simulink model "SIMULINK_PID_Tracking"  (R2023b)
settings: Solver=FixedStepAuto  StartTime=0.0  StopTime=sim_end_time  FixedStep=fixed_step_size  RelTol=1e-3
undefined symbols (not defined in the file): a, act_end, b, battery_threshold, bb, draw_gif, droneyeeUAV2_NUM, droneyeeUAV3_NUM, droneyeeUAV4_NUM, droneyeeUAV5_NUM, fixed_step_size, k, KD_x, KD_y, kd_z, KDD_x, KDD_y, KI_x, KI_y, ki_z, KII_x, KII_y, KP_x, KP_y, kp_z, KPP_x, KPP_y, lmt, omega, R, sim_end_time, uav10num, uav1num, uav2num, uav3num, uav4num, uav5num, uav6num, uav7num, uav8num, uav9num, UAV_NUM, Vel_Switch_1, Vel_Switch_10, Vel_Switch_11, Vel_Switch_12, Vel_Switch_13, Vel_Switch_14, Vel_Switch_15, Vel_Switch_16, Vel_Switch_17, Vel_Switch_18, Vel_Switch_19, Vel_Switch_2, Vel_Switch_20, Vel_Switch_3, Vel_Switch_4, Vel_Switch_5, Vel_Switch_6, Vel_Switch_7 ... (+12)
libraries: simulink x120, aerolibanimutils x1
(part 7 of 10)

== system SIMULINK_PID_Tracking/CMD_UAV/CMD3/Subsystem ==
  clock : Inport
  uavstates : Inport  Port=2
  Constant : Constant  Value=uav3num
  MATLAB Function : MATLAB Function  TreatAsAtomicUnit=on
  "xd " : Outport  VectorParamsAs1DForOutWhenUnconnected=off
  yd : Outport  Port=2  VectorParamsAs1DForOutWhenUnconnected=off
  zd : Outport  Port=3  VectorParamsAs1DForOutWhenUnconnected=off
  wires:
  uavstates/1 -> MATLAB Function/4(stas)
  [switch_flag] -> MATLAB Function/3(switch_flag)
  [avo_flag] -> MATLAB Function/7(avo_flag)
  [trj_flag] -> MATLAB Function/5(trj_flag)
  Constant/1 -> MATLAB Function/2(uavnum)
  [form_flag] -> MATLAB Function/6(form_flag)
  clock/1 -> MATLAB Function/1(timestamp)
  MATLAB Function/1(x_) -> "xd "/1
  MATLAB Function/2(y_) -> yd/1
  MATLAB Function/3(z_) -> zd/1

== system SIMULINK_PID_Tracking/CMD_UAV/CMD4/Subsystem ==
  clock : Inport
  uavstates : Inport  Port=2
  Constant : Constant  Value=uav4num
  MATLAB Function : MATLAB Function  TreatAsAtomicUnit=on
  "xd " : Outport  VectorParamsAs1DForOutWhenUnconnected=off
  yd : Outport  Port=2  VectorParamsAs1DForOutWhenUnconnected=off
  zd : Outport  Port=3  VectorParamsAs1DForOutWhenUnconnected=off
  wires:
  uavstates/1 -> MATLAB Function/4(stas)
  [switch_flag] -> MATLAB Function/3(switch_flag)
  [avo_flag] -> MATLAB Function/7(avo_flag)
  [trj_flag] -> MATLAB Function/5(trj_flag)
  Constant/1 -> MATLAB Function/2(uavnum)
  [form_flag] -> MATLAB Function/6(form_flag)
  clock/1 -> MATLAB Function/1(timestamp)
  MATLAB Function/1(x_) -> "xd "/1
  MATLAB Function/2(y_) -> yd/1
  MATLAB Function/3(z_) -> zd/1

== system SIMULINK_PID_Tracking/CMD_UAV/CMD5/Subsystem ==
  clock : Inport
  uavstates : Inport  Port=2
  Constant : Constant  Value=uav5num
  MATLAB Function : MATLAB Function  TreatAsAtomicUnit=on
  "xd " : Outport  VectorParamsAs1DForOutWhenUnconnected=off
  yd : Outport  Port=2  VectorParamsAs1DForOutWhenUnconnected=off
  zd : Outport  Port=3  VectorParamsAs1DForOutWhenUnconnected=off
  wires:
  uavstates/1 -> MATLAB Function/4(stas)
  [switch_flag] -> MATLAB Function/3(switch_flag)
  [avo_flag] -> MATLAB Function/7(avo_flag)
  [trj_flag] -> MATLAB Function/5(trj_flag)
  Constant/1 -> MATLAB Function/2(uavnum)
  [form_flag] -> MATLAB Function/6(form_flag)
  clock/1 -> MATLAB Function/1(timestamp)
  MATLAB Function/1(x_) -> "xd "/1
  MATLAB Function/2(y_) -> yd/1
  MATLAB Function/3(z_) -> zd/1

== system SIMULINK_PID_Tracking/CMD_UAV/CMD6/Subsystem ==
  clock : Inport
  uavstates : Inport  Port=2
  Constant : Constant  Value=uav6num
  MATLAB Function : MATLAB Function  TreatAsAtomicUnit=on
  "xd " : Outport  VectorParamsAs1DForOutWhenUnconnected=off
  yd : Outport  Port=2  VectorParamsAs1DForOutWhenUnconnected=off
  zd : Outport  Port=3  VectorParamsAs1DForOutWhenUnconnected=off
  wires:
  MATLAB Function/1(x_) -> "xd "/1
  MATLAB Function/2(y_) -> yd/1
  MATLAB Function/3(z_) -> zd/1
  clock/1 -> MATLAB Function/1(timestamp)
  Constant/1 -> MATLAB Function/2(uavnum)
  [switch_flag] -> MATLAB Function/3(switch_flag)
  uavstates/1 -> MATLAB Function/4(stas)
  [trj_flag] -> MATLAB Function/5(trj_flag)
  [form_flag] -> MATLAB Function/6(form_flag)
  [avo_flag] -> MATLAB Function/7(avo_flag)

== system SIMULINK_PID_Tracking/CMD_UAV/CMD7/Subsystem ==
  clock : Inport
  uavstates : Inport  Port=2
  Constant : Constant  Value=uav7num
  MATLAB Function : MATLAB Function  TreatAsAtomicUnit=on
  "xd " : Outport  VectorParamsAs1DForOutWhenUnconnected=off
  yd : Outport  Port=2  VectorParamsAs1DForOutWhenUnconnected=off
  zd : Outport  Port=3  VectorParamsAs1DForOutWhenUnconnected=off
  wires:
  uavstates/1 -> MATLAB Function/4(stas)
  [switch_flag] -> MATLAB Function/3(switch_flag)
  [avo_flag] -> MATLAB Function/7(avo_flag)
  [trj_flag] -> MATLAB Function/5(trj_flag)
  Constant/1 -> MATLAB Function/2(uavnum)
  [form_flag] -> MATLAB Function/6(form_flag)
  clock/1 -> MATLAB Function/1(timestamp)
  MATLAB Function/1(x_) -> "xd "/1
  MATLAB Function/2(y_) -> yd/1
  MATLAB Function/3(z_) -> zd/1

== system SIMULINK_PID_Tracking/CMD_UAV/CMD8/Subsystem ==
  clock : Inport
  uavstates : Inport  Port=2
  Constant : Constant  Value=uav8num
  MATLAB Function : MATLAB Function  TreatAsAtomicUnit=on
  "xd " : Outport  VectorParamsAs1DForOutWhenUnconnected=off
  yd : Outport  Port=2  VectorParamsAs1DForOutWhenUnconnected=off
  zd : Outport  Port=3  VectorParamsAs1DForOutWhenUnconnected=off
  wires:
  MATLAB Function/1(x_) -> "xd "/1
  MATLAB Function/2(y_) -> yd/1
  MATLAB Function/3(z_) -> zd/1
  clock/1 -> MATLAB Function/1(timestamp)
  Constant/1 -> MATLAB Function/2(uavnum)
  [switch_flag] -> MATLAB Function/3(switch_flag)
  uavstates/1 -> MATLAB Function/4(stas)
  [trj_flag] -> MATLAB Function/5(trj_flag)
  [form_flag] -> MATLAB Function/6(form_flag)
  [avo_flag] -> MATLAB Function/7(avo_flag)

== system SIMULINK_PID_Tracking/CMD_UAV/CMD9/Subsystem ==
  clock : Inport
  uavstates : Inport  Port=2
  Constant : Constant  Value=uav9num
  MATLAB Function : MATLAB Function  TreatAsAtomicUnit=on
  "xd " : Outport  VectorParamsAs1DForOutWhenUnconnected=off
  yd : Outport  Port=2  VectorParamsAs1DForOutWhenUnconnected=off
  zd : Outport  Port=3  VectorParamsAs1DForOutWhenUnconnected=off
  wires:
  uavstates/1 -> MATLAB Function/4(stas)
  [switch_flag] -> MATLAB Function/3(switch_flag)
  [avo_flag] -> MATLAB Function/7(avo_flag)
  [trj_flag] -> MATLAB Function/5(trj_flag)
  Constant/1 -> MATLAB Function/2(uavnum)
  [form_flag] -> MATLAB Function/6(form_flag)
  clock/1 -> MATLAB Function/1(timestamp)
  MATLAB Function/1(x_) -> "xd "/1
  MATLAB Function/2(y_) -> yd/1
  MATLAB Function/3(z_) -> zd/1

== system SIMULINK_PID_Tracking/CMD_car1/CMD1/Subsystem ==
  clock : Inport
  uavstates : Inport  Port=2
  Constant : Constant  Value=uav1num
  MATLAB Function : MATLAB Function  TreatAsAtomicUnit=on
  "xd " : Outport  VectorParamsAs1DForOutWhenUnconnected=off
  yd : Outport  Port=2  VectorParamsAs1DForOutWhenUnconnected=off
  zd : Outport  Port=3  VectorParamsAs1DForOutWhenUnconnected=off
  wires:
  MATLAB Function/1(x_) -> "xd "/1
  MATLAB Function/2(y_) -> yd/1
  MATLAB Function/3(z_) -> zd/1
  clock/1 -> MATLAB Function/1(timestamp)
  Constant/1 -> MATLAB Function/2(uavnum)
  [switch_flag] -> MATLAB Function/3(switch_flag)
  uavstates/1 -> MATLAB Function/4(stas)
  [trj_flag] -> MATLAB Function/5(trj_flag)
  [form_flag] -> MATLAB Function/6(form_flag)
  [avo_flag] -> MATLAB Function/7(avo_flag)

== system SIMULINK_PID_Tracking/CMD_car1/CMD10/Subsystem ==
  clock : Inport
  uavstates : Inport  Port=2
  Constant : Constant  Value=uav10num
  Goto : Goto  Commented=on  GotoTag=trj_flag  TagVisibility=global
  Goto1 : Goto  Commented=on  GotoTag=form_flag  TagVisibility=global
  Goto2 : Goto  Commented=on  GotoTag=avo_flag  TagVisibility=global
  MATLAB Function : MATLAB Function  TreatAsAtomicUnit=on
  轨迹 : Constant  Commented=on
  避障 : Constant  Commented=on  Value=0
  队形 : Constant  Commented=on
  "xd " : Outport  VectorParamsAs1DForOutWhenUnconnected=off
  yd : Outport  Port=2  VectorParamsAs1DForOutWhenUnconnected=off
  zd : Outport  Port=3  VectorParamsAs1DForOutWhenUnconnected=off
  wires:
  MATLAB Function/1(x_) -> "xd "/1
  MATLAB Function/2(y_) -> yd/1
  MATLAB Function/3(z_) -> zd/1
  clock/1 -> MATLAB Function/1(timestamp)
  Constant/1 -> MATLAB Function/2(uavnum)
  [switch_flag] -> MATLAB Function/3(switch_flag)
  uavstates/1 -> MATLAB Function/4(stas)
  轨迹/1 -> Goto/1
  队形/1 -> Goto1/1
  避障/1 -> Goto2/1
  [trj_flag] -> MATLAB Function/5(trj_flag)
  [form_flag] -> MATLAB Function/6(form_flag)
  [avo_flag] -> MATLAB Function/7(avo_flag)

== system SIMULINK_PID_Tracking/CMD_car1/CMD2/Subsystem ==
  clock : Inport
  uavstates : Inport  Port=2
  Constant : Constant  Value=uav2num
  MATLAB Function : MATLAB Function  TreatAsAtomicUnit=on
  "xd " : Outport  VectorParamsAs1DForOutWhenUnconnected=off
  yd : Outport  Port=2  VectorParamsAs1DForOutWhenUnconnected=off
  zd : Outport  Port=3  VectorParamsAs1DForOutWhenUnconnected=off
  wires:
  uavstates/1 -> MATLAB Function/4(stas)
  [switch_flag] -> MATLAB Function/3(switch_flag)
  [avo_flag] -> MATLAB Function/7(avo_flag)
  [trj_flag] -> MATLAB Function/5(trj_flag)
  Constant/1 -> MATLAB Function/2(uavnum)
  [form_flag] -> MATLAB Function/6(form_flag)
  clock/1 -> MATLAB Function/1(timestamp)
  MATLAB Function/1(x_) -> "xd "/1
  MATLAB Function/3(z_) -> zd/1
  MATLAB Function/2(y_) -> yd/1

== system SIMULINK_PID_Tracking/CMD_car1/CMD3/Subsystem ==
  clock : Inport
  uavstates : Inport  Port=2
  Constant : Constant  Value=uav3num
  MATLAB Function : MATLAB Function  TreatAsAtomicUnit=on
  "xd " : Outport  VectorParamsAs1DForOutWhenUnconnected=off
  yd : Outport  Port=2  VectorParamsAs1DForOutWhenUnconnected=off
  zd : Outport  Port=3  VectorParamsAs1DForOutWhenUnconnected=off
  wires:
  uavstates/1 -> MATLAB Function/4(stas)
  [switch_flag] -> MATLAB Function/3(switch_flag)
  [avo_flag] -> MATLAB Function/7(avo_flag)
  [trj_flag] -> MATLAB Function/5(trj_flag)
  Constant/1 -> MATLAB Function/2(uavnum)
  [form_flag] -> MATLAB Function/6(form_flag)
  clock/1 -> MATLAB Function/1(timestamp)
  MATLAB Function/1(x_) -> "xd "/1
  MATLAB Function/2(y_) -> yd/1
  MATLAB Function/3(z_) -> zd/1

== system SIMULINK_PID_Tracking/CMD_car1/CMD4/Subsystem ==
  clock : Inport
  uavstates : Inport  Port=2
  Constant : Constant  Value=uav4num
  MATLAB Function : MATLAB Function  TreatAsAtomicUnit=on
  "xd " : Outport  VectorParamsAs1DForOutWhenUnconnected=off
  yd : Outport  Port=2  VectorParamsAs1DForOutWhenUnconnected=off
  zd : Outport  Port=3  VectorParamsAs1DForOutWhenUnconnected=off
  wires:
  uavstates/1 -> MATLAB Function/4(stas)
  [switch_flag] -> MATLAB Function/3(switch_flag)
  [avo_flag] -> MATLAB Function/7(avo_flag)
  [trj_flag] -> MATLAB Function/5(trj_flag)
  Constant/1 -> MATLAB Function/2(uavnum)
  [form_flag] -> MATLAB Function/6(form_flag)
  clock/1 -> MATLAB Function/1(timestamp)
  MATLAB Function/1(x_) -> "xd "/1
  MATLAB Function/2(y_) -> yd/1
  MATLAB Function/3(z_) -> zd/1

== system SIMULINK_PID_Tracking/CMD_car1/CMD5/Subsystem ==
  clock : Inport
  uavstates : Inport  Port=2
  Constant : Constant  Value=uav5num
  MATLAB Function : MATLAB Function  TreatAsAtomicUnit=on
  "xd " : Outport  VectorParamsAs1DForOutWhenUnconnected=off
  yd : Outport  Port=2  VectorParamsAs1DForOutWhenUnconnected=off
  zd : Outport  Port=3  VectorParamsAs1DForOutWhenUnconnected=off
  wires:
  uavstates/1 -> MATLAB Function/4(stas)
  [switch_flag] -> MATLAB Function/3(switch_flag)
  [avo_flag] -> MATLAB Function/7(avo_flag)
  [trj_flag] -> MATLAB Function/5(trj_flag)
  Constant/1 -> MATLAB Function/2(uavnum)
  [form_flag] -> MATLAB Function/6(form_flag)
  clock/1 -> MATLAB Function/1(timestamp)
  MATLAB Function/1(x_) -> "xd "/1
  MATLAB Function/2(y_) -> yd/1
  MATLAB Function/3(z_) -> zd/1

== system SIMULINK_PID_Tracking/CMD_car1/CMD6/Subsystem ==
  clock : Inport
  uavstates : Inport  Port=2
  Constant : Constant  Value=uav6num
  MATLAB Function : MATLAB Function  TreatAsAtomicUnit=on
  "xd " : Outport  VectorParamsAs1DForOutWhenUnconnected=off
  yd : Outport  Port=2  VectorParamsAs1DForOutWhenUnconnected=off
  zd : Outport  Port=3  VectorParamsAs1DForOutWhenUnconnected=off
  wires:
  MATLAB Function/1(x_) -> "xd "/1
  MATLAB Function/2(y_) -> yd/1
  MATLAB Function/3(z_) -> zd/1
  clock/1 -> MATLAB Function/1(timestamp)
  Constant/1 -> MATLAB Function/2(uavnum)
  [switch_flag] -> MATLAB Function/3(switch_flag)
  uavstates/1 -> MATLAB Function/4(stas)
  [trj_flag] -> MATLAB Function/5(trj_flag)
  [form_flag] -> MATLAB Function/6(form_flag)
  [avo_flag] -> MATLAB Function/7(avo_flag)

== system SIMULINK_PID_Tracking/CMD_car1/CMD7/Subsystem ==
  clock : Inport
  uavstates : Inport  Port=2
  Constant : Constant  Value=uav7num
  MATLAB Function : MATLAB Function  TreatAsAtomicUnit=on
  "xd " : Outport  VectorParamsAs1DForOutWhenUnconnected=off
  yd : Outport  Port=2  VectorParamsAs1DForOutWhenUnconnected=off
  zd : Outport  Port=3  VectorParamsAs1DForOutWhenUnconnected=off
  wires:
  uavstates/1 -> MATLAB Function/4(stas)
  [switch_flag] -> MATLAB Function/3(switch_flag)
  [avo_flag] -> MATLAB Function/7(avo_flag)
  [trj_flag] -> MATLAB Function/5(trj_flag)
  Constant/1 -> MATLAB Function/2(uavnum)
  [form_flag] -> MATLAB Function/6(form_flag)
  clock/1 -> MATLAB Function/1(timestamp)
  MATLAB Function/1(x_) -> "xd "/1
  MATLAB Function/2(y_) -> yd/1
  MATLAB Function/3(z_) -> zd/1

== system SIMULINK_PID_Tracking/CMD_car1/CMD8/Subsystem ==
  clock : Inport
  uavstates : Inport  Port=2
  Constant : Constant  Value=uav8num
  MATLAB Function : MATLAB Function  TreatAsAtomicUnit=on
  "xd " : Outport  VectorParamsAs1DForOutWhenUnconnected=off
  yd : Outport  Port=2  VectorParamsAs1DForOutWhenUnconnected=off
  zd : Outport  Port=3  VectorParamsAs1DForOutWhenUnconnected=off
  wires:
  MATLAB Function/1(x_) -> "xd "/1
  MATLAB Function/2(y_) -> yd/1
  MATLAB Function/3(z_) -> zd/1
  clock/1 -> MATLAB Function/1(timestamp)
  Constant/1 -> MATLAB Function/2(uavnum)
  [switch_flag] -> MATLAB Function/3(switch_flag)
  uavstates/1 -> MATLAB Function/4(stas)
  [trj_flag] -> MATLAB Function/5(trj_flag)
  [form_flag] -> MATLAB Function/6(form_flag)
  [avo_flag] -> MATLAB Function/7(avo_flag)

== system SIMULINK_PID_Tracking/CMD_car1/CMD9/Subsystem ==
  clock : Inport
  uavstates : Inport  Port=2
  Constant : Constant  Value=uav9num
  MATLAB Function : MATLAB Function  TreatAsAtomicUnit=on
  "xd " : Outport  VectorParamsAs1DForOutWhenUnconnected=off
  yd : Outport  Port=2  VectorParamsAs1DForOutWhenUnconnected=off
  zd : Outport  Port=3  VectorParamsAs1DForOutWhenUnconnected=off
  wires:
  uavstates/1 -> MATLAB Function/4(stas)
  [switch_flag] -> MATLAB Function/3(switch_flag)
  [avo_flag] -> MATLAB Function/7(avo_flag)
  [trj_flag] -> MATLAB Function/5(trj_flag)
  Constant/1 -> MATLAB Function/2(uavnum)
  [form_flag] -> MATLAB Function/6(form_flag)
  clock/1 -> MATLAB Function/1(timestamp)
  MATLAB Function/1(x_) -> "xd "/1
  MATLAB Function/2(y_) -> yd/1
  MATLAB Function/3(z_) -> zd/1

== system SIMULINK_PID_Tracking/control system_UAV/Baseline Controller1/Heading controller ==
  yaw_e (rad) : Inport
  yaw_d. (rad) : Inport  Port=2
  Integrator Limited : Integrator  Commented=on  LimitOutput=on  UpperSaturationLimit=0.3  LowerSaturationLimit=-0.3
  Ki : Gain  Commented=on  Gain=0.01
  Sum1 : Sum  Inputs=|-+
  Sum2 : Sum  Inputs=|++
  proportional control gain - yaw : Gain  Gain=0.2
  yaw_rate_d. (rad/s) : Outport  VectorParamsAs1DForOutWhenUnconnected=off
  wires:
  Sum1/1 -> Ki/1, proportional control gain - yaw/1
  yaw_e (rad)/1 -> Sum1/1
  yaw_d. (rad)/1 -> Sum1/2
  proportional control gain - yaw/1 -> Sum2/1
  Integrator Limited/1 -> Sum2/2
  Ki/1 -> Integrator Limited/1
  Sum2/1 -> yaw_rate_d. (rad/s)/1

== system SIMULINK_PID_Tracking/control system_UAV/Baseline Controller1/Height controller  ==
  Z_d. (m) : Inport
  Z_e (m) : Inport  Port=2
  V_z : Inport  Port=3
  Discrete Derivative1 : simulink/Discrete/Discrete Derivative  gainval=1.0  ICPrevScaledInput=0.0  OutMin=[]  OutMax=[]  OutDataType=fixdt(1, 16)  OutScaling=2^-10  DoSatur=off
  Integrator Limited : Integrator  LimitOutput=on  UpperSaturationLimit=0.1  LowerSaturationLimit=-0.1
  Kd : Gain  Gain=kd_z
  Ki : Gain  Gain=ki_z
  Kp : Gain  Gain=kp_z
  Sum2 : Sum  Inputs=+++
  Sum3 : Sum  Inputs=|-+
  Z_velocity_d (m/s) : Outport  VectorParamsAs1DForOutWhenUnconnected=off
  wires:
  Sum3/1 -> Discrete Derivative1/1, Ki/1, Kp/1
  Z_e (m)/1 -> Sum3/1
  Discrete Derivative1/1 -> Kd/1
  Sum2/1 -> Z_velocity_d (m/s)/1
  Kp/1 -> Sum2/2
  Kd/1 -> Sum2/3
  Ki/1 -> Integrator Limited/1
  Integrator Limited/1 -> Sum2/1
  Z_d. (m)/1 -> Sum3/2

== system SIMULINK_PID_Tracking/control system_UAV/Baseline Controller1/Position controller ==
  X_e (m) : Inport
  Y_e (m) : Inport  Port=2
  X_d (m) : Inport  Port=3
  Y_d (m) : Inport  Port=4
  Discrete Derivative1 : simulink/Discrete/Discrete Derivative  gainval=1.0  ICPrevScaledInput=0.0  OutMin=[]  OutMax=[]  OutDataType=fixdt(1, 16)  OutScaling=2^-10  DoSatur=off
  Discrete Derivative2 : simulink/Discrete/Discrete Derivative  gainval=1.0  ICPrevScaledInput=0.0  OutMin=[]  OutMax=[]  OutDataType=fixdt(1, 16)  OutScaling=2^-10  DoSatur=off
  Integrator Limited : Integrator  LimitOutput=on  UpperSaturationLimit=0.4  LowerSaturationLimit=-0.4
  Integrator Limited1 : Integrator  LimitOutput=on  UpperSaturationLimit=0.4  LowerSaturationLimit=-0.4
  Kd : Gain  Gain=KD_x
  Kd1 : Gain  Gain=KD_y
  Kp : Gain  Gain=KP_x
  Kp1 : Gain  Gain=KI_x
  Kp2 : Gain  Gain=KP_y
  Kp3 : Gain  Gain=KI_y
  Mux : Mux  Inputs=2
  Sum2 : Sum  Inputs=+++
  Sum3 : Sum  Inputs=|-+
  Sum5 : Sum  Inputs=+++
  Sum6 : Sum  Inputs=|-+
  uxy : Outport  VectorParamsAs1DForOutWhenUnconnected=off
  wires:
  Sum5/1 -> Mux/2
  Discrete Derivative1/1 -> Kd/1
  Kp2/1 -> Sum5/2
  Sum3/1 -> Discrete Derivative1/1, Kp/1, Kp1/1
  Discrete Derivative2/1 -> Kd1/1
  X_d (m)/1 -> Sum3/2
  Integrator Limited/1 -> Sum2/1
  Y_d (m)/1 -> Sum6/2
  Kp3/1 -> Integrator Limited1/1
  Kp1/1 -> Integrator Limited/1
  Kd1/1 -> Sum5/3
  Mux/1 -> uxy/1
  Kp/1 -> Sum2/2
  X_e (m)/1 -> Sum3/1
  Integrator Limited1/1 -> Sum5/1
  Sum2/1 -> Mux/1
  Kd/1 -> Sum2/3
  Y_e (m)/1 -> Sum6/1
  Sum6/1 -> Discrete Derivative2/1, Kp2/1, Kp3/1

== system SIMULINK_PID_Tracking/control system_UAV/Baseline Controller10/Heading controller ==
  yaw_e (rad) : Inport
  yaw_d. (rad) : Inport  Port=2
  Integrator Limited : Integrator  Commented=on  LimitOutput=on  UpperSaturationLimit=0.3  LowerSaturationLimit=-0.3
  Ki : Gain  Commented=on  Gain=0.01
  Sum1 : Sum  Inputs=|-+
  Sum2 : Sum  Inputs=|++
  proportional control gain - yaw : Gain  Gain=0.2
  yaw_rate_d. (rad/s) : Outport  VectorParamsAs1DForOutWhenUnconnected=off
  wires:
  Sum1/1 -> Ki/1, proportional control gain - yaw/1
  yaw_e (rad)/1 -> Sum1/1
  yaw_d. (rad)/1 -> Sum1/2
  proportional control gain - yaw/1 -> Sum2/1
  Integrator Limited/1 -> Sum2/2
  Ki/1 -> Integrator Limited/1
  Sum2/1 -> yaw_rate_d. (rad/s)/1

== system SIMULINK_PID_Tracking/control system_UAV/Baseline Controller10/Height controller  ==
  Z_d. (m) : Inport
  Z_e (m) : Inport  Port=2
  V_z : Inport  Port=3
  Discrete Derivative1 : simulink/Discrete/Discrete Derivative  gainval=1.0  ICPrevScaledInput=0.0  OutMin=[]  OutMax=[]  OutDataType=fixdt(1, 16)  OutScaling=2^-10  DoSatur=off
  Integrator Limited : Integrator  LimitOutput=on  UpperSaturationLimit=0.1  LowerSaturationLimit=-0.1
  Kd : Gain  Gain=kd_z
  Ki : Gain  Gain=ki_z
  Kp : Gain  Gain=kp_z
  Sum2 : Sum  Inputs=+++
  Sum3 : Sum  Inputs=|-+
  Z_velocity_d (m/s) : Outport  VectorParamsAs1DForOutWhenUnconnected=off
  wires:
  Sum3/1 -> Discrete Derivative1/1, Ki/1, Kp/1
  Z_e (m)/1 -> Sum3/1
  Discrete Derivative1/1 -> Kd/1
  Sum2/1 -> Z_velocity_d (m/s)/1
  Kp/1 -> Sum2/2
  Kd/1 -> Sum2/3
  Ki/1 -> Integrator Limited/1
  Integrator Limited/1 -> Sum2/1
  Z_d. (m)/1 -> Sum3/2

== system SIMULINK_PID_Tracking/control system_UAV/Baseline Controller10/Position controller ==
  X_e (m) : Inport
  Y_e (m) : Inport  Port=2
  X_d (m) : Inport  Port=3
  Y_d (m) : Inport  Port=4
  Discrete Derivative1 : simulink/Discrete/Discrete Derivative  gainval=1.0  ICPrevScaledInput=0.0  OutMin=[]  OutMax=[]  OutDataType=fixdt(1, 16)  OutScaling=2^-10  DoSatur=off
  Discrete Derivative2 : simulink/Discrete/Discrete Derivative  gainval=1.0  ICPrevScaledInput=0.0  OutMin=[]  OutMax=[]  OutDataType=fixdt(1, 16)  OutScaling=2^-10  DoSatur=off
  Integrator Limited : Integrator  LimitOutput=on  UpperSaturationLimit=0.5  LowerSaturationLimit=-0.5
  Integrator Limited1 : Integrator  LimitOutput=on  UpperSaturationLimit=0.5  LowerSaturationLimit=-0.5
  Kd : Gain  Gain=KD_x
  Kd1 : Gain  Gain=KD_y
  Kp : Gain  Gain=KP_x
  Kp1 : Gain  Gain=KI_x
  Kp2 : Gain  Gain=KP_y
  Kp3 : Gain  Gain=KI_y
  Mux : Mux  Inputs=2
  Scope : Scope
  Scope1 : Scope
  Sum2 : Sum  Inputs=+++
  Sum3 : Sum  Inputs=|-+
  Sum5 : Sum  Inputs=+++
  Sum6 : Sum  Inputs=|-+
  uxy : Outport  VectorParamsAs1DForOutWhenUnconnected=off
  wires:
  X_e (m)/1 -> Sum3/1
  Integrator Limited/1 -> Sum2/1
  Sum2/1 -> Mux/1, Scope/1
  Kp1/1 -> Integrator Limited/1
  Kp/1 -> Sum2/2
  Kp2/1 -> Sum5/2
  Y_e (m)/1 -> Sum6/1
  Integrator Limited1/1 -> Sum5/1
  Sum5/1 -> Mux/2, Scope1/1
  Kp3/1 -> Integrator Limited1/1
  Mux/1 -> uxy/1
  X_d (m)/1 -> Sum3/2
  Discrete Derivative1/1 -> Kd/1
  Sum3/1 -> Discrete Derivative1/1, Kp/1, Kp1/1
  Y_d (m)/1 -> Sum6/2
  Sum6/1 -> Discrete Derivative2/1, Kp2/1, Kp3/1
  Kd1/1 -> Sum5/3
  Discrete Derivative2/1 -> Kd1/1
  Kd/1 -> Sum2/3

== system SIMULINK_PID_Tracking/control system_UAV/Baseline Controller2/Heading controller ==
  yaw_e (rad) : Inport
  yaw_d. (rad) : Inport  Port=2
  Integrator Limited : Integrator  Commented=on  LimitOutput=on  UpperSaturationLimit=0.3  LowerSaturationLimit=-0.3
  Ki : Gain  Commented=on  Gain=0.01
  Sum1 : Sum  Inputs=|-+
  Sum2 : Sum  Inputs=|++
  proportional control gain - yaw : Gain  Gain=0.2
  yaw_rate_d. (rad/s) : Outport  VectorParamsAs1DForOutWhenUnconnected=off
  wires:
  Sum2/1 -> yaw_rate_d. (rad/s)/1
  Ki/1 -> Integrator Limited/1
  Integrator Limited/1 -> Sum2/2
  proportional control gain - yaw/1 -> Sum2/1
  yaw_d. (rad)/1 -> Sum1/2
  yaw_e (rad)/1 -> Sum1/1
  Sum1/1 -> proportional control gain - yaw/1, Ki/1

== system SIMULINK_PID_Tracking/control system_UAV/Baseline Controller2/Height controller  ==
  Z_d. (m) : Inport
  Z_e (m) : Inport  Port=2
  V_z : Inport  Port=3
  Discrete Derivative1 : simulink/Discrete/Discrete Derivative  gainval=1.0  ICPrevScaledInput=0.0  OutMin=[]  OutMax=[]  OutDataType=fixdt(1, 16)  OutScaling=2^-10  DoSatur=off
  Integrator Limited : Integrator  LimitOutput=on  UpperSaturationLimit=0.1  LowerSaturationLimit=-0.1
  Kd : Gain  Gain=kd_z
  Ki : Gain  Gain=ki_z
  Kp : Gain  Gain=kp_z
  Sum2 : Sum  Inputs=+++
  Sum3 : Sum  Inputs=|-+
  Z_velocity_d (m/s) : Outport  VectorParamsAs1DForOutWhenUnconnected=off
  wires:
  Sum3/1 -> Discrete Derivative1/1, Ki/1, Kp/1
  Z_e (m)/1 -> Sum3/1
  Discrete Derivative1/1 -> Kd/1
  Sum2/1 -> Z_velocity_d (m/s)/1
  Kp/1 -> Sum2/2
  Kd/1 -> Sum2/3
  Ki/1 -> Integrator Limited/1
  Integrator Limited/1 -> Sum2/1
  Z_d. (m)/1 -> Sum3/2

== system SIMULINK_PID_Tracking/control system_UAV/Baseline Controller2/Position controller ==
  X_e (m) : Inport
  Y_e (m) : Inport  Port=2
  X_d (m) : Inport  Port=3
  Y_d (m) : Inport  Port=4
  Discrete Derivative1 : simulink/Discrete/Discrete Derivative  gainval=1.0  ICPrevScaledInput=0.0  OutMin=[]  OutMax=[]  OutDataType=fixdt(1, 16)  OutScaling=2^-10  DoSatur=off
  Discrete Derivative2 : simulink/Discrete/Discrete Derivative  gainval=1.0  ICPrevScaledInput=0.0  OutMin=[]  OutMax=[]  OutDataType=fixdt(1, 16)  OutScaling=2^-10  DoSatur=off
  Integrator Limited : Integrator  LimitOutput=on  UpperSaturationLimit=0.4  LowerSaturationLimit=-0.4
  Integrator Limited1 : Integrator  LimitOutput=on  UpperSaturationLimit=0.4  LowerSaturationLimit=-0.4
  Kd : Gain  Gain=KD_x
  Kd1 : Gain  Gain=KD_y
  Kp : Gain  Gain=KP_x
  Kp1 : Gain  Gain=KI_x
  Kp2 : Gain  Gain=KP_y
  Kp3 : Gain  Gain=KI_y
  Mux : Mux  Inputs=2
  Sum2 : Sum  Inputs=+++
  Sum3 : Sum  Inputs=|-+
  Sum5 : Sum  Inputs=+++
  Sum6 : Sum  Inputs=|-+
  uxy : Outport  VectorParamsAs1DForOutWhenUnconnected=off
  wires:
  Discrete Derivative2/1 -> Kd1/1
  Kd1/1 -> Sum5/3
  Sum6/1 -> Discrete Derivative2/1, Kp2/1, Kp3/1
  Y_d (m)/1 -> Sum6/2
  Kd/1 -> Sum2/3
  Discrete Derivative1/1 -> Kd/1
  Sum3/1 -> Discrete Derivative1/1, Kp1/1, Kp/1
  X_d (m)/1 -> Sum3/2
  Mux/1 -> uxy/1
  Kp3/1 -> Integrator Limited1/1
  Integrator Limited1/1 -> Sum5/1
  Y_e (m)/1 -> Sum6/1
  Kp2/1 -> Sum5/2
  Kp/1 -> Sum2/2
  Kp1/1 -> Integrator Limited/1
  Integrator Limited/1 -> Sum2/1
  X_e (m)/1 -> Sum3/1
  Sum2/1 -> Mux/1
  Sum5/1 -> Mux/2

== system SIMULINK_PID_Tracking/control system_UAV/Baseline Controller3/Heading controller ==
  yaw_e (rad) : Inport
  yaw_d. (rad) : Inport  Port=2
  Integrator Limited : Integrator  Commented=on  LimitOutput=on  UpperSaturationLimit=0.3  LowerSaturationLimit=-0.3
  Ki : Gain  Commented=on  Gain=0.01
  Sum1 : Sum  Inputs=|-+
  Sum2 : Sum  Inputs=|++
  proportional control gain - yaw : Gain  Gain=0.2
  yaw_rate_d. (rad/s) : Outport  VectorParamsAs1DForOutWhenUnconnected=off
  wires:
  Sum1/1 -> Ki/1, proportional control gain - yaw/1
  yaw_e (rad)/1 -> Sum1/1
  yaw_d. (rad)/1 -> Sum1/2
  proportional control gain - yaw/1 -> Sum2/1
  Integrator Limited/1 -> Sum2/2
  Ki/1 -> Integrator Limited/1
  Sum2/1 -> yaw_rate_d. (rad/s)/1

== system SIMULINK_PID_Tracking/control system_UAV/Baseline Controller3/Height controller  ==
  Z_d. (m) : Inport
  Z_e (m) : Inport  Port=2
  V_z : Inport  Port=3
  Discrete Derivative1 : simulink/Discrete/Discrete Derivative  gainval=1.0  ICPrevScaledInput=0.0  OutMin=[]  OutMax=[]  OutDataType=fixdt(1, 16)  OutScaling=2^-10  DoSatur=off
  Integrator Limited : Integrator  LimitOutput=on  UpperSaturationLimit=0.1  LowerSaturationLimit=-0.1
  Kd : Gain  Gain=kd_z
  Ki : Gain  Gain=ki_z
  Kp : Gain  Gain=kp_z
  Sum2 : Sum  Inputs=+++
  Sum3 : Sum  Inputs=|-+
  Z_velocity_d (m/s) : Outport  VectorParamsAs1DForOutWhenUnconnected=off
  wires:
  Sum3/1 -> Discrete Derivative1/1, Ki/1, Kp/1
  Z_e (m)/1 -> Sum3/1
  Discrete Derivative1/1 -> Kd/1
  Sum2/1 -> Z_velocity_d (m/s)/1
  Kp/1 -> Sum2/2
  Kd/1 -> Sum2/3
  Ki/1 -> Integrator Limited/1
  Integrator Limited/1 -> Sum2/1
  Z_d. (m)/1 -> Sum3/2

== system SIMULINK_PID_Tracking/control system_UAV/Baseline Controller3/Position controller ==
  X_e (m) : Inport
  Y_e (m) : Inport  Port=2
  X_d (m) : Inport  Port=3
  Y_d (m) : Inport  Port=4
  Discrete Derivative1 : simulink/Discrete/Discrete Derivative  gainval=1.0  ICPrevScaledInput=0.0  OutMin=[]  OutMax=[]  OutDataType=fixdt(1, 16)  OutScaling=2^-10  DoSatur=off
  Discrete Derivative2 : simulink/Discrete/Discrete Derivative  gainval=1.0  ICPrevScaledInput=0.0  OutMin=[]  OutMax=[]  OutDataType=fixdt(1, 16)  OutScaling=2^-10  DoSatur=off
  Integrator Limited : Integrator  LimitOutput=on  UpperSaturationLimit=0.5  LowerSaturationLimit=-0.5
  Integrator Limited1 : Integrator  LimitOutput=on  UpperSaturationLimit=0.5  LowerSaturationLimit=-0.5
  Kd : Gain  Gain=KD_x
  Kd1 : Gain  Gain=KD_y
  Kp : Gain  Gain=KP_x
  Kp1 : Gain  Gain=KI_x
  Kp2 : Gain  Gain=KP_y
  Kp3 : Gain  Gain=KI_y
  Mux : Mux  Inputs=2
  Sum2 : Sum  Inputs=+++
  Sum3 : Sum  Inputs=|-+
  Sum5 : Sum  Inputs=+++
  Sum6 : Sum  Inputs=|-+
  uxy : Outport  VectorParamsAs1DForOutWhenUnconnected=off
  wires:
  X_e (m)/1 -> Sum3/1
  Integrator Limited/1 -> Sum2/1
  Kp1/1 -> Integrator Limited/1
  Kp/1 -> Sum2/2
  Kp2/1 -> Sum5/2
  Y_e (m)/1 -> Sum6/1
  Integrator Limited1/1 -> Sum5/1
  Kp3/1 -> Integrator Limited1/1
  Mux/1 -> uxy/1
  X_d (m)/1 -> Sum3/2
  Discrete Derivative1/1 -> Kd/1
  Kd/1 -> Sum2/3
  Sum3/1 -> Discrete Derivative1/1, Kp/1, Kp1/1
  Y_d (m)/1 -> Sum6/2
  Sum6/1 -> Discrete Derivative2/1, Kp2/1, Kp3/1
  Kd1/1 -> Sum5/3
  Discrete Derivative2/1 -> Kd1/1
  Sum2/1 -> Mux/1
  Sum5/1 -> Mux/2

== system SIMULINK_PID_Tracking/control system_UAV/Baseline Controller4/Heading controller ==
  yaw_e (rad) : Inport
  yaw_d. (rad) : Inport  Port=2
  Integrator Limited : Integrator  Commented=on  LimitOutput=on  UpperSaturationLimit=0.3  LowerSaturationLimit=-0.3
  Ki : Gain  Commented=on  Gain=0.01
  Sum1 : Sum  Inputs=|-+
  Sum2 : Sum  Inputs=|++
  proportional control gain - yaw : Gain  Gain=0.2
  yaw_rate_d. (rad/s) : Outport  VectorParamsAs1DForOutWhenUnconnected=off
  wires:
  Sum2/1 -> yaw_rate_d. (rad/s)/1
  Ki/1 -> Integrator Limited/1
  Integrator Limited/1 -> Sum2/2
  proportional control gain - yaw/1 -> Sum2/1
  yaw_d. (rad)/1 -> Sum1/2
  yaw_e (rad)/1 -> Sum1/1
  Sum1/1 -> proportional control gain - yaw/1, Ki/1

== system SIMULINK_PID_Tracking/control system_UAV/Baseline Controller4/Height controller  ==
  Z_d. (m) : Inport
  Z_e (m) : Inport  Port=2
  V_z : Inport  Port=3
  Discrete Derivative1 : simulink/Discrete/Discrete Derivative  gainval=1.0  ICPrevScaledInput=0.0  OutMin=[]  OutMax=[]  OutDataType=fixdt(1, 16)  OutScaling=2^-10  DoSatur=off
  Integrator Limited : Integrator  LimitOutput=on  UpperSaturationLimit=0.1  LowerSaturationLimit=-0.1
  Kd : Gain  Gain=kd_z
  Ki : Gain  Gain=ki_z
  Kp : Gain  Gain=kp_z
  Sum2 : Sum  Inputs=+++
  Sum3 : Sum  Inputs=|-+
  Z_velocity_d (m/s) : Outport  VectorParamsAs1DForOutWhenUnconnected=off
  wires:
  Sum3/1 -> Discrete Derivative1/1, Ki/1, Kp/1
  Z_e (m)/1 -> Sum3/1
  Discrete Derivative1/1 -> Kd/1
  Sum2/1 -> Z_velocity_d (m/s)/1
  Kp/1 -> Sum2/2
  Kd/1 -> Sum2/3
  Ki/1 -> Integrator Limited/1
  Integrator Limited/1 -> Sum2/1
  Z_d. (m)/1 -> Sum3/2

== system SIMULINK_PID_Tracking/control system_UAV/Baseline Controller4/Position controller ==
  X_e (m) : Inport
  Y_e (m) : Inport  Port=2
  X_d (m) : Inport  Port=3
  Y_d (m) : Inport  Port=4
  Discrete Derivative1 : simulink/Discrete/Discrete Derivative  gainval=1.0  ICPrevScaledInput=0.0  OutMin=[]  OutMax=[]  OutDataType=fixdt(1, 16)  OutScaling=2^-10  DoSatur=off
  Discrete Derivative2 : simulink/Discrete/Discrete Derivative  gainval=1.0  ICPrevScaledInput=0.0  OutMin=[]  OutMax=[]  OutDataType=fixdt(1, 16)  OutScaling=2^-10  DoSatur=off
  Integrator Limited : Integrator  LimitOutput=on  UpperSaturationLimit=0.5  LowerSaturationLimit=-0.5
  Integrator Limited1 : Integrator  LimitOutput=on  UpperSaturationLimit=0.5  LowerSaturationLimit=-0.5
  Kd : Gain  Gain=KD_x
  Kd1 : Gain  Gain=KD_y
  Kp : Gain  Gain=KP_x
  Kp1 : Gain  Gain=KI_x
  Kp2 : Gain  Gain=KP_y
  Kp3 : Gain  Gain=KI_y
  Mux : Mux  Inputs=2
  Sum2 : Sum  Inputs=+++
  Sum3 : Sum  Inputs=|-+
  Sum5 : Sum  Inputs=+++
  Sum6 : Sum  Inputs=|-+
  uxy : Outport  VectorParamsAs1DForOutWhenUnconnected=off
  wires:
  Discrete Derivative2/1 -> Kd1/1
  Kd1/1 -> Sum5/3
  Sum6/1 -> Discrete Derivative2/1, Kp3/1, Kp2/1
  Y_d (m)/1 -> Sum6/2
  Sum3/1 -> Discrete Derivative1/1, Kp1/1, Kp/1
  Kd/1 -> Sum2/3
  Discrete Derivative1/1 -> Kd/1
  X_d (m)/1 -> Sum3/2
  Mux/1 -> uxy/1
  Kp3/1 -> Integrator Limited1/1
  Integrator Limited1/1 -> Sum5/1
  Y_e (m)/1 -> Sum6/1
  Kp2/1 -> Sum5/2
  Kp/1 -> Sum2/2
  Kp1/1 -> Integrator Limited/1
  Integrator Limited/1 -> Sum2/1
  X_e (m)/1 -> Sum3/1
  Sum5/1 -> Mux/2
  Sum2/1 -> Mux/1

== system SIMULINK_PID_Tracking/control system_UAV/Baseline Controller5/Heading controller ==
  yaw_e (rad) : Inport
  yaw_d. (rad) : Inport  Port=2
  Integrator Limited : Integrator  Commented=on  LimitOutput=on  UpperSaturationLimit=0.3  LowerSaturationLimit=-0.3
  Ki : Gain  Commented=on  Gain=0.01
  Sum1 : Sum  Inputs=|-+
  Sum2 : Sum  Inputs=|++
  proportional control gain - yaw : Gain  Gain=0.2
  yaw_rate_d. (rad/s) : Outport  VectorParamsAs1DForOutWhenUnconnected=off
  wires:
  Sum1/1 -> Ki/1, proportional control gain - yaw/1
  yaw_e (rad)/1 -> Sum1/1
  yaw_d. (rad)/1 -> Sum1/2
  proportional control gain - yaw/1 -> Sum2/1
  Integrator Limited/1 -> Sum2/2
  Ki/1 -> Integrator Limited/1
  Sum2/1 -> yaw_rate_d. (rad/s)/1

== system SIMULINK_PID_Tracking/control system_UAV/Baseline Controller5/Height controller  ==
  Z_d. (m) : Inport
  Z_e (m) : Inport  Port=2
  V_z : Inport  Port=3
  Discrete Derivative1 : simulink/Discrete/Discrete Derivative  gainval=1.0  ICPrevScaledInput=0.0  OutMin=[]  OutMax=[]  OutDataType=fixdt(1, 16)  OutScaling=2^-10  DoSatur=off
  Integrator Limited : Integrator  LimitOutput=on  UpperSaturationLimit=0.1  LowerSaturationLimit=-0.1
  Kd : Gain  Gain=kd_z
  Ki : Gain  Gain=ki_z
  Kp : Gain  Gain=kp_z
  Sum2 : Sum  Inputs=+++
  Sum3 : Sum  Inputs=|-+
  Z_velocity_d (m/s) : Outport  VectorParamsAs1DForOutWhenUnconnected=off
  wires:
  Sum3/1 -> Discrete Derivative1/1, Ki/1, Kp/1
  Z_e (m)/1 -> Sum3/1
  Discrete Derivative1/1 -> Kd/1
  Sum2/1 -> Z_velocity_d (m/s)/1
  Kp/1 -> Sum2/2
  Kd/1 -> Sum2/3
  Ki/1 -> Integrator Limited/1
  Integrator Limited/1 -> Sum2/1
  Z_d. (m)/1 -> Sum3/2

== system SIMULINK_PID_Tracking/control system_UAV/Baseline Controller5/Position controller ==
  X_e (m) : Inport
  Y_e (m) : Inport  Port=2
  X_d (m) : Inport  Port=3
  Y_d (m) : Inport  Port=4
  Discrete Derivative1 : simulink/Discrete/Discrete Derivative  gainval=1.0  ICPrevScaledInput=0.0  OutMin=[]  OutMax=[]  OutDataType=fixdt(1, 16)  OutScaling=2^-10  DoSatur=off
  Discrete Derivative2 : simulink/Discrete/Discrete Derivative  gainval=1.0  ICPrevScaledInput=0.0  OutMin=[]  OutMax=[]  OutDataType=fixdt(1, 16)  OutScaling=2^-10  DoSatur=off
  Integrator Limited : Integrator  LimitOutput=on  UpperSaturationLimit=0.5  LowerSaturationLimit=-0.5
  Integrator Limited1 : Integrator  LimitOutput=on  UpperSaturationLimit=0.5  LowerSaturationLimit=-0.5
  Kd : Gain  Gain=KD_x
  Kd1 : Gain  Gain=KD_y
  Kp : Gain  Gain=KP_x
  Kp1 : Gain  Gain=KI_x
  Kp2 : Gain  Gain=KP_y
  Kp3 : Gain  Gain=KI_y
  Mux : Mux  Inputs=2
  Scope : Scope
  Scope1 : Scope
  Sum2 : Sum  Inputs=+++
  Sum3 : Sum  Inputs=|-+
  Sum5 : Sum  Inputs=+++
  Sum6 : Sum  Inputs=|-+
  uxy : Outport  VectorParamsAs1DForOutWhenUnconnected=off
  wires:
  X_e (m)/1 -> Sum3/1
  Integrator Limited/1 -> Sum2/1
  Sum2/1 -> Mux/1, Scope/1
  Kp1/1 -> Integrator Limited/1
  Kp/1 -> Sum2/2
  Kp2/1 -> Sum5/2
  Y_e (m)/1 -> Sum6/1
  Integrator Limited1/1 -> Sum5/1
  Sum5/1 -> Mux/2, Scope1/1
  Kp3/1 -> Integrator Limited1/1
  Mux/1 -> uxy/1
  X_d (m)/1 -> Sum3/2
  Discrete Derivative1/1 -> Kd/1
  Sum3/1 -> Discrete Derivative1/1, Kp/1, Kp1/1
  Y_d (m)/1 -> Sum6/2
  Sum6/1 -> Discrete Derivative2/1, Kp2/1, Kp3/1
  Kd1/1 -> Sum5/3
  Discrete Derivative2/1 -> Kd1/1
  Kd/1 -> Sum2/3

== system SIMULINK_PID_Tracking/control system_UAV/Baseline Controller6/Heading controller ==
  yaw_e (rad) : Inport
  yaw_d. (rad) : Inport  Port=2
  Integrator Limited : Integrator  Commented=on  LimitOutput=on  UpperSaturationLimit=0.3  LowerSaturationLimit=-0.3
  Ki : Gain  Commented=on  Gain=0.01
  Sum1 : Sum  Inputs=|-+
  Sum2 : Sum  Inputs=|++
  proportional control gain - yaw : Gain  Gain=0.2
  yaw_rate_d. (rad/s) : Outport  VectorParamsAs1DForOutWhenUnconnected=off
  wires:
  Sum1/1 -> Ki/1, proportional control gain - yaw/1
  yaw_e (rad)/1 -> Sum1/1
  yaw_d. (rad)/1 -> Sum1/2
  proportional control gain - yaw/1 -> Sum2/1
  Integrator Limited/1 -> Sum2/2
  Ki/1 -> Integrator Limited/1
  Sum2/1 -> yaw_rate_d. (rad/s)/1

== system SIMULINK_PID_Tracking/control system_UAV/Baseline Controller6/Height controller  ==
  Z_d. (m) : Inport
  Z_e (m) : Inport  Port=2
  V_z : Inport  Port=3
  Discrete Derivative1 : simulink/Discrete/Discrete Derivative  gainval=1.0  ICPrevScaledInput=0.0  OutMin=[]  OutMax=[]  OutDataType=fixdt(1, 16)  OutScaling=2^-10  DoSatur=off
  Integrator Limited : Integrator  LimitOutput=on  UpperSaturationLimit=0.1  LowerSaturationLimit=-0.1
  Kd : Gain  Gain=kd_z
  Ki : Gain  Gain=ki_z
  Kp : Gain  Gain=kp_z
  Sum2 : Sum  Inputs=+++
  Sum3 : Sum  Inputs=|-+
  Z_velocity_d (m/s) : Outport  VectorParamsAs1DForOutWhenUnconnected=off
  wires:
  Sum3/1 -> Discrete Derivative1/1, Ki/1, Kp/1
  Z_e (m)/1 -> Sum3/1
  Discrete Derivative1/1 -> Kd/1
  Sum2/1 -> Z_velocity_d (m/s)/1
  Kp/1 -> Sum2/2
  Kd/1 -> Sum2/3
  Ki/1 -> Integrator Limited/1
  Integrator Limited/1 -> Sum2/1
  Z_d. (m)/1 -> Sum3/2

== system SIMULINK_PID_Tracking/control system_UAV/Baseline Controller6/Position controller ==
  X_e (m) : Inport
  Y_e (m) : Inport  Port=2
  X_d (m) : Inport  Port=3
  Y_d (m) : Inport  Port=4
  Discrete Derivative1 : simulink/Discrete/Discrete Derivative  gainval=1.0  ICPrevScaledInput=0.0  OutMin=[]  OutMax=[]  OutDataType=fixdt(1, 16)  OutScaling=2^-10  DoSatur=off
  Discrete Derivative2 : simulink/Discrete/Discrete Derivative  gainval=1.0  ICPrevScaledInput=0.0  OutMin=[]  OutMax=[]  OutDataType=fixdt(1, 16)  OutScaling=2^-10  DoSatur=off
  Integrator Limited : Integrator  LimitOutput=on  UpperSaturationLimit=0.5  LowerSaturationLimit=-0.5
  Integrator Limited1 : Integrator  LimitOutput=on  UpperSaturationLimit=0.5  LowerSaturationLimit=-0.5
  Kd : Gain  Gain=KD_x
  Kd1 : Gain  Gain=KD_y
  Kp : Gain  Gain=KP_x
  Kp1 : Gain  Gain=KI_x
  Kp2 : Gain  Gain=KP_y
  Kp3 : Gain  Gain=KI_y
  Mux : Mux  Inputs=2
  Scope : Scope
  Scope1 : Scope
  Sum2 : Sum  Inputs=+++
  Sum3 : Sum  Inputs=|-+
  Sum5 : Sum  Inputs=+++
  Sum6 : Sum  Inputs=|-+
  uxy : Outport  VectorParamsAs1DForOutWhenUnconnected=off
  wires:
  X_e (m)/1 -> Sum3/1
  Integrator Limited/1 -> Sum2/1
  Sum2/1 -> Mux/1, Scope/1
  Kp1/1 -> Integrator Limited/1
  Kp/1 -> Sum2/2
  Kp2/1 -> Sum5/2
  Y_e (m)/1 -> Sum6/1
  Integrator Limited1/1 -> Sum5/1
  Sum5/1 -> Mux/2, Scope1/1
  Kp3/1 -> Integrator Limited1/1
  Mux/1 -> uxy/1
  X_d (m)/1 -> Sum3/2
  Discrete Derivative1/1 -> Kd/1
  Sum3/1 -> Discrete Derivative1/1, Kp/1, Kp1/1
  Y_d (m)/1 -> Sum6/2
  Sum6/1 -> Discrete Derivative2/1, Kp2/1, Kp3/1
  Kd1/1 -> Sum5/3
  Discrete Derivative2/1 -> Kd1/1
  Kd/1 -> Sum2/3

== system SIMULINK_PID_Tracking/control system_UAV/Baseline Controller7/Heading controller ==
  yaw_e (rad) : Inport
  yaw_d. (rad) : Inport  Port=2
  Integrator Limited : Integrator  Commented=on  LimitOutput=on  UpperSaturationLimit=0.3  LowerSaturationLimit=-0.3
  Ki : Gain  Commented=on  Gain=0.01
  Sum1 : Sum  Inputs=|-+
  Sum2 : Sum  Inputs=|++
  proportional control gain - yaw : Gain  Gain=0.2
  yaw_rate_d. (rad/s) : Outport  VectorParamsAs1DForOutWhenUnconnected=off
  wires:
  Sum1/1 -> Ki/1, proportional control gain - yaw/1
  yaw_e (rad)/1 -> Sum1/1
  yaw_d. (rad)/1 -> Sum1/2
  proportional control gain - yaw/1 -> Sum2/1
  Integrator Limited/1 -> Sum2/2
  Ki/1 -> Integrator Limited/1
  Sum2/1 -> yaw_rate_d. (rad/s)/1

== system SIMULINK_PID_Tracking/control system_UAV/Baseline Controller7/Height controller  ==
  Z_d. (m) : Inport
  Z_e (m) : Inport  Port=2
  V_z : Inport  Port=3
  Discrete Derivative1 : simulink/Discrete/Discrete Derivative  gainval=1.0  ICPrevScaledInput=0.0  OutMin=[]  OutMax=[]  OutDataType=fixdt(1, 16)  OutScaling=2^-10  DoSatur=off
  Integrator Limited : Integrator  LimitOutput=on  UpperSaturationLimit=0.1  LowerSaturationLimit=-0.1
  Kd : Gain  Gain=kd_z
  Ki : Gain  Gain=ki_z
  Kp : Gain  Gain=kp_z
  Sum2 : Sum  Inputs=+++
  Sum3 : Sum  Inputs=|-+
  Z_velocity_d (m/s) : Outport  VectorParamsAs1DForOutWhenUnconnected=off
  wires:
  Sum3/1 -> Discrete Derivative1/1, Ki/1, Kp/1
  Z_e (m)/1 -> Sum3/1
  Discrete Derivative1/1 -> Kd/1
  Sum2/1 -> Z_velocity_d (m/s)/1
  Kp/1 -> Sum2/2
  Kd/1 -> Sum2/3
  Ki/1 -> Integrator Limited/1
  Integrator Limited/1 -> Sum2/1
  Z_d. (m)/1 -> Sum3/2

== system SIMULINK_PID_Tracking/control system_UAV/Baseline Controller7/Position controller ==
  X_e (m) : Inport
  Y_e (m) : Inport  Port=2
  X_d (m) : Inport  Port=3
  Y_d (m) : Inport  Port=4
  Discrete Derivative1 : simulink/Discrete/Discrete Derivative  gainval=1.0  ICPrevScaledInput=0.0  OutMin=[]  OutMax=[]  OutDataType=fixdt(1, 16)  OutScaling=2^-10  DoSatur=off
  Discrete Derivative2 : simulink/Discrete/Discrete Derivative  gainval=1.0  ICPrevScaledInput=0.0  OutMin=[]  OutMax=[]  OutDataType=fixdt(1, 16)  OutScaling=2^-10  DoSatur=off
  Integrator Limited : Integrator  LimitOutput=on  UpperSaturationLimit=0.5  LowerSaturationLimit=-0.5
  Integrator Limited1 : Integrator  LimitOutput=on  UpperSaturationLimit=0.5  LowerSaturationLimit=-0.5
  Kd : Gain  Gain=KD_x
  Kd1 : Gain  Gain=KD_y
  Kp : Gain  Gain=KP_x
  Kp1 : Gain  Gain=KI_x
  Kp2 : Gain  Gain=KP_y
  Kp3 : Gain  Gain=KI_y
  Mux : Mux  Inputs=2
  Scope : Scope
  Scope1 : Scope
  Sum2 : Sum  Inputs=+++
  Sum3 : Sum  Inputs=|-+
  Sum5 : Sum  Inputs=+++
  Sum6 : Sum  Inputs=|-+
  uxy : Outport  VectorParamsAs1DForOutWhenUnconnected=off
  wires:
  X_e (m)/1 -> Sum3/1
  Integrator Limited/1 -> Sum2/1
  Sum2/1 -> Mux/1, Scope/1
  Kp1/1 -> Integrator Limited/1
  Kp/1 -> Sum2/2
  Kp2/1 -> Sum5/2
  Y_e (m)/1 -> Sum6/1
  Integrator Limited1/1 -> Sum5/1
  Sum5/1 -> Mux/2, Scope1/1
  Kp3/1 -> Integrator Limited1/1
  Mux/1 -> uxy/1
  X_d (m)/1 -> Sum3/2
  Discrete Derivative1/1 -> Kd/1
  Sum3/1 -> Discrete Derivative1/1, Kp/1, Kp1/1
  Y_d (m)/1 -> Sum6/2
  Sum6/1 -> Discrete Derivative2/1, Kp2/1, Kp3/1
  Kd1/1 -> Sum5/3
  Discrete Derivative2/1 -> Kd1/1
  Kd/1 -> Sum2/3

== system SIMULINK_PID_Tracking/control system_UAV/Baseline Controller8/Heading controller ==
  yaw_e (rad) : Inport
  yaw_d. (rad) : Inport  Port=2
  Integrator Limited : Integrator  Commented=on  LimitOutput=on  UpperSaturationLimit=0.3  LowerSaturationLimit=-0.3
  Ki : Gain  Commented=on  Gain=0.01
  Sum1 : Sum  Inputs=|-+
  Sum2 : Sum  Inputs=|++
  proportional control gain - yaw : Gain  Gain=0.2
  yaw_rate_d. (rad/s) : Outport  VectorParamsAs1DForOutWhenUnconnected=off
  wires:
  Sum1/1 -> Ki/1, proportional control gain - yaw/1
  yaw_e (rad)/1 -> Sum1/1
  yaw_d. (rad)/1 -> Sum1/2
  proportional control gain - yaw/1 -> Sum2/1
  Integrator Limited/1 -> Sum2/2
  Ki/1 -> Integrator Limited/1
  Sum2/1 -> yaw_rate_d. (rad/s)/1

== system SIMULINK_PID_Tracking/control system_UAV/Baseline Controller8/Height controller  ==
  Z_d. (m) : Inport
  Z_e (m) : Inport  Port=2
  V_z : Inport  Port=3
  Discrete Derivative1 : simulink/Discrete/Discrete Derivative  gainval=1.0  ICPrevScaledInput=0.0  OutMin=[]  OutMax=[]  OutDataType=fixdt(1, 16)  OutScaling=2^-10  DoSatur=off
  Integrator Limited : Integrator  LimitOutput=on  UpperSaturationLimit=0.1  LowerSaturationLimit=-0.1
  Kd : Gain  Gain=kd_z
  Ki : Gain  Gain=ki_z
  Kp : Gain  Gain=kp_z
  Sum2 : Sum  Inputs=+++
  Sum3 : Sum  Inputs=|-+
  Z_velocity_d (m/s) : Outport  VectorParamsAs1DForOutWhenUnconnected=off
  wires:
  Sum3/1 -> Discrete Derivative1/1, Ki/1, Kp/1
  Z_e (m)/1 -> Sum3/1
  Discrete Derivative1/1 -> Kd/1
  Sum2/1 -> Z_velocity_d (m/s)/1
  Kp/1 -> Sum2/2
  Kd/1 -> Sum2/3
  Ki/1 -> Integrator Limited/1
  Integrator Limited/1 -> Sum2/1
  Z_d. (m)/1 -> Sum3/2

== system SIMULINK_PID_Tracking/control system_UAV/Baseline Controller8/Position controller ==
  X_e (m) : Inport
  Y_e (m) : Inport  Port=2
  X_d (m) : Inport  Port=3
  Y_d (m) : Inport  Port=4
  Discrete Derivative1 : simulink/Discrete/Discrete Derivative  gainval=1.0  ICPrevScaledInput=0.0  OutMin=[]  OutMax=[]  OutDataType=fixdt(1, 16)  OutScaling=2^-10  DoSatur=off
  Discrete Derivative2 : simulink/Discrete/Discrete Derivative  gainval=1.0  ICPrevScaledInput=0.0  OutMin=[]  OutMax=[]  OutDataType=fixdt(1, 16)  OutScaling=2^-10  DoSatur=off
  Integrator Limited : Integrator  LimitOutput=on  UpperSaturationLimit=0.5  LowerSaturationLimit=-0.5
  Integrator Limited1 : Integrator  LimitOutput=on  UpperSaturationLimit=0.5  LowerSaturationLimit=-0.5
  Kd : Gain  Gain=KD_x
  Kd1 : Gain  Gain=KD_y
  Kp : Gain  Gain=KP_x
  Kp1 : Gain  Gain=KI_x
  Kp2 : Gain  Gain=KP_y
  Kp3 : Gain  Gain=KI_y
  Mux : Mux  Inputs=2
  Scope : Scope
  Scope1 : Scope
  Sum2 : Sum  Inputs=+++
  Sum3 : Sum  Inputs=|-+
  Sum5 : Sum  Inputs=+++
  Sum6 : Sum  Inputs=|-+
  uxy : Outport  VectorParamsAs1DForOutWhenUnconnected=off
  wires:
  X_e (m)/1 -> Sum3/1
  Integrator Limited/1 -> Sum2/1
  Sum2/1 -> Mux/1, Scope/1
  Kp1/1 -> Integrator Limited/1
  Kp/1 -> Sum2/2
  Kp2/1 -> Sum5/2
  Y_e (m)/1 -> Sum6/1
  Integrator Limited1/1 -> Sum5/1
  Sum5/1 -> Mux/2, Scope1/1
  Kp3/1 -> Integrator Limited1/1
  Mux/1 -> uxy/1
  X_d (m)/1 -> Sum3/2
  Discrete Derivative1/1 -> Kd/1
  Sum3/1 -> Discrete Derivative1/1, Kp/1, Kp1/1
  Y_d (m)/1 -> Sum6/2
  Sum6/1 -> Discrete Derivative2/1, Kp2/1, Kp3/1
  Kd1/1 -> Sum5/3
  Discrete Derivative2/1 -> Kd1/1
  Kd/1 -> Sum2/3

== system SIMULINK_PID_Tracking/control system_UAV/Baseline Controller9/Heading controller ==
  yaw_e (rad) : Inport
  yaw_d. (rad) : Inport  Port=2
  Integrator Limited : Integrator  Commented=on  LimitOutput=on  UpperSaturationLimit=0.3  LowerSaturationLimit=-0.3
  Ki : Gain  Commented=on  Gain=0.01
  Sum1 : Sum  Inputs=|-+
  Sum2 : Sum  Inputs=|++
  proportional control gain - yaw : Gain  Gain=0.2
  yaw_rate_d. (rad/s) : Outport  VectorParamsAs1DForOutWhenUnconnected=off
  wires:
  Sum1/1 -> Ki/1, proportional control gain - yaw/1
  yaw_e (rad)/1 -> Sum1/1
  yaw_d. (rad)/1 -> Sum1/2
  proportional control gain - yaw/1 -> Sum2/1
  Integrator Limited/1 -> Sum2/2
  Ki/1 -> Integrator Limited/1
  Sum2/1 -> yaw_rate_d. (rad/s)/1

== system SIMULINK_PID_Tracking/control system_UAV/Baseline Controller9/Height controller  ==
  Z_d. (m) : Inport
  Z_e (m) : Inport  Port=2
  V_z : Inport  Port=3
  Discrete Derivative1 : simulink/Discrete/Discrete Derivative  gainval=1.0  ICPrevScaledInput=0.0  OutMin=[]  OutMax=[]  OutDataType=fixdt(1, 16)  OutScaling=2^-10  DoSatur=off
  Integrator Limited : Integrator  LimitOutput=on  UpperSaturationLimit=0.1  LowerSaturationLimit=-0.1
  Kd : Gain  Gain=kd_z
  Ki : Gain  Gain=ki_z
  Kp : Gain  Gain=kp_z
  Sum2 : Sum  Inputs=+++
  Sum3 : Sum  Inputs=|-+
  Z_velocity_d (m/s) : Outport  VectorParamsAs1DForOutWhenUnconnected=off
  wires:
  Sum3/1 -> Discrete Derivative1/1, Ki/1, Kp/1
  Z_e (m)/1 -> Sum3/1
  Discrete Derivative1/1 -> Kd/1
  Sum2/1 -> Z_velocity_d (m/s)/1
  Kp/1 -> Sum2/2
  Kd/1 -> Sum2/3
  Ki/1 -> Integrator Limited/1
  Integrator Limited/1 -> Sum2/1
  Z_d. (m)/1 -> Sum3/2

== system SIMULINK_PID_Tracking/control system_UAV/Baseline Controller9/Position controller ==
  X_e (m) : Inport
  Y_e (m) : Inport  Port=2
  X_d (m) : Inport  Port=3
  Y_d (m) : Inport  Port=4
  Discrete Derivative1 : simulink/Discrete/Discrete Derivative  gainval=1.0  ICPrevScaledInput=0.0  OutMin=[]  OutMax=[]  OutDataType=fixdt(1, 16)  OutScaling=2^-10  DoSatur=off
  Discrete Derivative2 : simulink/Discrete/Discrete Derivative  gainval=1.0  ICPrevScaledInput=0.0  OutMin=[]  OutMax=[]  OutDataType=fixdt(1, 16)  OutScaling=2^-10  DoSatur=off
  Integrator Limited : Integrator  LimitOutput=on  UpperSaturationLimit=0.5  LowerSaturationLimit=-0.5
  Integrator Limited1 : Integrator  LimitOutput=on  UpperSaturationLimit=0.5  LowerSaturationLimit=-0.5
  Kd : Gain  Gain=KD_x
  Kd1 : Gain  Gain=KD_y
  Kp : Gain  Gain=KP_x
  Kp1 : Gain  Gain=KI_x
  Kp2 : Gain  Gain=KP_y
  Kp3 : Gain  Gain=KI_y
  Mux : Mux  Inputs=2
  Scope : Scope
  Scope1 : Scope
  Sum2 : Sum  Inputs=+++
  Sum3 : Sum  Inputs=|-+
  Sum5 : Sum  Inputs=+++
  Sum6 : Sum  Inputs=|-+
  uxy : Outport  VectorParamsAs1DForOutWhenUnconnected=off
  wires:
  X_e (m)/1 -> Sum3/1
  Integrator Limited/1 -> Sum2/1
  Sum2/1 -> Mux/1, Scope/1
  Kp1/1 -> Integrator Limited/1
  Kp/1 -> Sum2/2
  Kp2/1 -> Sum5/2
  Y_e (m)/1 -> Sum6/1
  Integrator Limited1/1 -> Sum5/1
  Sum5/1 -> Mux/2, Scope1/1
  Kp3/1 -> Integrator Limited1/1
  Mux/1 -> uxy/1
  X_d (m)/1 -> Sum3/2
  Discrete Derivative1/1 -> Kd/1
  Sum3/1 -> Discrete Derivative1/1, Kp/1, Kp1/1
  Y_d (m)/1 -> Sum6/2
  Sum6/1 -> Discrete Derivative2/1, Kp2/1, Kp3/1
  Kd1/1 -> Sum5/3
  Discrete Derivative2/1 -> Kd1/1
  Kd/1 -> Sum2/3

== system SIMULINK_PID_Tracking/control system_car1/Baseline Controller1/Heading controller ==
  yaw_e (rad) : Inport
  yaw_d. (rad) : Inport  Port=2
  Integrator Limited : Integrator  Commented=on  LimitOutput=on  UpperSaturationLimit=0.3  LowerSaturationLimit=-0.3
  Ki : Gain  Commented=on  Gain=0.01
  Sum1 : Sum  Inputs=|-+
  Sum2 : Sum  Inputs=|++
  proportional control gain - yaw : Gain  Gain=0.2
  yaw_rate_d. (rad/s) : Outport  VectorParamsAs1DForOutWhenUnconnected=off
  wires:
  Sum1/1 -> Ki/1, proportional control gain - yaw/1
  yaw_e (rad)/1 -> Sum1/1
  yaw_d. (rad)/1 -> Sum1/2
  proportional control gain - yaw/1 -> Sum2/1
  Integrator Limited/1 -> Sum2/2
  Ki/1 -> Integrator Limited/1
  Sum2/1 -> yaw_rate_d. (rad/s)/1

== system SIMULINK_PID_Tracking/control system_car1/Baseline Controller1/Height controller  ==
  Z_d. (m) : Inport
  Z_e (m) : Inport  Port=2
  V_z : Inport  Port=3
  Discrete Derivative1 : simulink/Discrete/Discrete Derivative  gainval=1.0  ICPrevScaledInput=0.0  OutMin=[]  OutMax=[]  OutDataType=fixdt(1, 16)  OutScaling=2^-10  DoSatur=off
  Integrator Limited : Integrator  LimitOutput=on  UpperSaturationLimit=0.1  LowerSaturationLimit=-0.1
  Kd : Gain  Gain=kd_z
  Ki : Gain  Gain=ki_z
  Kp : Gain  Gain=kp_z
  Sum2 : Sum  Inputs=+++
  Sum3 : Sum  Inputs=|-+
  Z_velocity_d (m/s) : Outport  VectorParamsAs1DForOutWhenUnconnected=off
  wires:
  Sum3/1 -> Discrete Derivative1/1, Ki/1, Kp/1
  Z_e (m)/1 -> Sum3/1
  Discrete Derivative1/1 -> Kd/1
  Sum2/1 -> Z_velocity_d (m/s)/1
  Kp/1 -> Sum2/2
  Kd/1 -> Sum2/3
  Ki/1 -> Integrator Limited/1
  Integrator Limited/1 -> Sum2/1
  Z_d. (m)/1 -> Sum3/2
